simulink model "teste_controlador18a"  (R2018a)
settings: Solver=VariableStepAuto  StartTime=0.0  StopTime=30  FixedStep=0.0001  RelTol=1e-6
InitFcn:
  | J = 0.916e-6;
  | B = 0.66e-6;
  | a0 = 0.738e-12;
  | a1 = 0.198e-10;
libraries: simulink x1
settings Model: Creator=easylab  LastModifiedBy=thiag
settings SFSimCC: SimUseLocalCustomCode=on
settings RTWCC: RTWUseLocalCustomCode=on

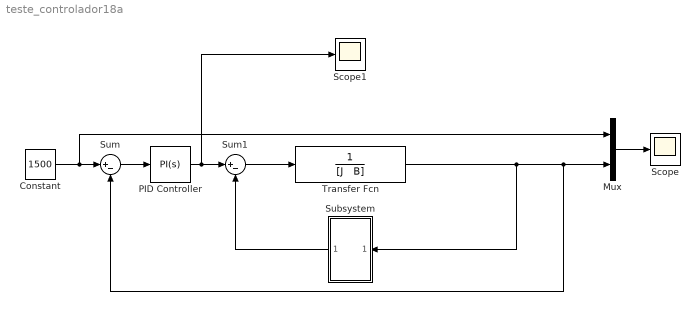
== system teste_controlador18a ==
  Constant : Constant  Value=1500
  Mux : Mux  Inputs=2
  PID Controller : simulink/Continuous/PID Controller  Controller=PI  TimeDomain=Continuous-time  SampleTime=-1  IntegratorMethod=Forward Euler  FilterMethod=Forward Euler  Form=Parallel  UseFilter=on  ControllerParametersSource=internal  P=1.63918032306973e-06  I=1.85695310261092e-06  D=0  N=100  InitialConditionSource=internal  InitialConditionForIntegrator=0  InitialConditionForFilter=0  ExternalReset=none  LimitOutput=off  UpperSaturationLimit=inf  LowerSaturationLimit=-inf  LinearizeAsGain=on  AntiWindupMode=none  Kb=1  TrackingMode=off  Kt=1  PParamMin=[]  PParamMax=[]  IParamMin=[]  IParamMax=[]  DParamMin=[]  DParamMax=[]  NParamMin=[]  NParamMax=[]  KbParamMin=[]  KbParamMax=[]  KtParamMin=[]  KtParamMax=[]  POutMin=[]  POutMax=[]  IOutMin=[]  IOutMax=[]  DOutMin=[]  DOutMax=[]  NOutMin=[]  NOutMax=[]  KbOutMin=[]  KbOutMax=[]  KtOutMin=[]  KtOutMax=[]  IntegratorOutMin=[]  IntegratorOutMax=[]  FilterOutMin=[]  FilterOutMax=[]  SumOutMin=[]  SumOutMax=[]  SumI1OutMin=[]  SumI1OutMax=[]  SumI2OutMin=[]  SumI2OutMax=[]  SumI3OutMin=[]  SumI3OutMax=[]  SumDOutMin=[]  SumDOutMax=[]  SaturationOutMin=[]  SaturationOutMax=[]  IntegratorContinuousStateAttributes=''  IntegratorStateMustResolveToSignalObject=off  IntegratorRTWStateStorageClass=Auto  FilterContinuousStateAttributes=''  FilterStateMustResolveToSignalObject=off  FilterRTWStateStorageClass=Auto  DifferentiatorICPrevScaledInput=0  DifferentiatorOutMin=[]  DifferentiatorOutMax=[]  FilterDiffOutCoefMin=[]  FilterDiffOutCoefMax=[]  SumDenOutMin=[]  SumDenOutMax=[]  SumNumOutMin=[]  SumNumOutMax=[]  ReciprocalOutMin=[]  ReciprocalOutMax=[]  DivideOutMin=[]  DivideOutMax=[]  TunerSelectOption=Transfer Function Based (PID Tuner App)
  Scope : Scope
  Scope1 : Scope
  Subsystem : Subsystem
  Sum : Sum  Inputs=|+-
  Sum1 : Sum  Inputs=|+-
  Transfer Fcn : TransferFcn  Denominator="[J   B]"
  wires:
  Sum1/1 -> Transfer Fcn/1
  Transfer Fcn/1 -> Sum/2, Mux/2, Subsystem/1(In1)
  Sum/1 -> PID Controller/1
  PID Controller/1 -> Scope1/1, Sum1/1
  Constant/1 -> Mux/1, Sum/1
  Mux/1 -> Scope/1
  Subsystem/1(Out1) -> Sum1/2

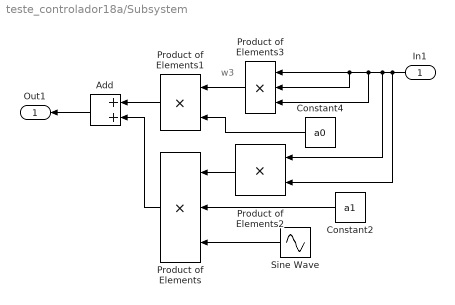
== system teste_controlador18a/Subsystem ==
  note: w3
  In1 : Inport
  Add : Sum
  Constant2 : Constant  Value=a1
  Constant4 : Constant  Value=a0
  Product of Elements : Product  Inputs=3
  Product of Elements1 : Product
  Product of Elements2 : Product
  Product of Elements3 : Product  Inputs=3
  Sine Wave : Sin  Amplitude=92  Bias=100  Frequency=2*pi*(1/0.67)  SampleTime=0
  Out1 : Outport
  wires:
  Constant4/1 -> Product of Elements1/2
  Product of Elements2/1 -> Product of Elements/1
  Constant2/1 -> Product of Elements/2
  Product of Elements1/1 -> Add/1
  In1/1 -> Product of Elements2/2, Product of Elements2/1, Product of Elements3/3, Product of Elements3/2, Product of Elements3/1
  Sine Wave/1 -> Product of Elements/3
  Product of Elements/1 -> Add/2
  Product of Elements3/1 -> Product of Elements1/1
  Add/1 -> Out1/1
